simulink model "Scenario_PlusJunction_TrafficLights"  (R2021a)
settings: Solver=VariableStepAuto  StartTime=0.0  StopTime=10.0  RelTol=1e-3
model workspace (MAT data in the model file):
  Kz_dif = Simulink.Parameter
  Kz_dif.Value = Simulink.data.Expression
  Kz_dif.Value.ExpressionString = " L_dif / (Lc + ds)"
  Kz_dif.DataType = 'auto'
  Kz_dif.Dimensions = -1
  Kz_il = Simulink.Parameter
  Kz_il.Value = Simulink.data.Expression
  Kz_il.Value.ExpressionString = " L_il / (Lc + ds)"
  Kz_il.DataType = 'auto'
  Kz_il.Dimensions = -1
  Kz_ir = Simulink.Parameter
  Kz_ir.Value = Simulink.data.Expression
  Kz_ir.Value.ExpressionString = " L_ir / (Lc + ds)"
  Kz_ir.DataType = 'auto'
  Kz_ir.Dimensions = -1
  Kz_is = Simulink.Parameter
  Kz_is.Value = Simulink.data.Expression
  Kz_is.Value.ExpressionString = " L_is / (Lc + ds)"
  Kz_is.DataType = 'auto'
  Kz_is.Dimensions = -1
  Kz_long = Simulink.Parameter
  Kz_long.Value = Simulink.data.Expression
  Kz_long.Value.ExpressionString = " L_long / (Lc + ds)"
  Kz_long.Description = 'Segmentkapazität (wie viele autos passen hinein)'
  Kz_long.DataType = 'auto'
  Kz_long.Dimensions = -1
  Kz_pre = Simulink.Parameter
  Kz_pre.Value = Simulink.data.Expression
  Kz_pre.Value.ExpressionString = " L_pre / (Lc + ds)"
  Kz_pre.DataType = 'auto'
  Kz_pre.Dimensions = -1
  L_dif = Simulink.Parameter
  L_dif.Value = Simulink.data.Expression
  L_dif.Value.ExpressionString = "L_long-L_pre"
  L_dif.Description = 'Differenz zwischen Abbiegerspurlänge und normaler straßenlänge'
  L_dif.DataType = 'auto'
  L_dif.Dimensions = -1
  L_il = Simulink.Parameter
  L_il.Value = 30
  L_il.Description = 'Länge der innenkreuzungssegments, das linksabbieger durchqueren'
  L_il.DataType = 'auto'
  L_il.Dimensions = [1 1]
  L_ir = Simulink.Parameter
  L_ir.Value = 23
  L_ir.Description = 'Länge der innenkreuzungssegments, das rechtsabbieger durchqueren'
  L_ir.DataType = 'auto'
  L_ir.Dimensions = [1 1]
  L_is = Simulink.Parameter
  L_is.Value = 35
  L_is.Description = 'Länge der innenkreuzungssegments, das geradeausfahrer durchqueren'
  L_is.DataType = 'auto'
  L_is.Dimensions = [1 1]
  L_long = Simulink.Parameter
  L_long.Value = 52.8
  L_long.Description = 'Langes straßensegment  (52.8 meter)'
  L_long.DataType = 'auto'
  L_long.Dimensions = [1 1]
  L_pre = Simulink.Parameter
  L_pre.Value = 20
  L_pre.Description = 'Länge der Abbiegespuren'
  L_pre.DataType = 'auto'
  L_pre.Dimensions = [1 1]
  Lc = Simulink.Parameter
  Lc.Value = 4.4
  Lc.Description = 'Länge eines autos'
  Lc.DataType = 'auto'
  Lc.Dimensions = [1 1]
  Rk = Simulink.Parameter
  Rk.Value = Simulink.data.Expression
  Rk.Value.ExpressionString = " 1 / (Lc / v)"
  Rk.Description = 'Flussrate zwischen den Kanten (bei speed v)'
  Rk.DataType = 'auto'
  Rk.Dimensions = -1
  Tz_dif = Simulink.Parameter
  Tz_dif.Value = Simulink.data.Expression
  Tz_dif.Value.ExpressionString = " L_dif / v"
  Tz_dif.DataType = 'auto'
  Tz_dif.Dimensions = -1
  Tz_il = Simulink.Parameter
  Tz_il.Value = Simulink.data.Expression
  Tz_il.Value.ExpressionString = " L_il / v"
  Tz_il.DataType = 'auto'
  Tz_il.Dimensions = -1
  Tz_ir = Simulink.Parameter
  Tz_ir.Value = Simulink.data.Expression
  Tz_ir.Value.ExpressionString = " L_ir / v"
  Tz_ir.DataType = 'auto'
  Tz_ir.Dimensions = -1
  Tz_is = Simulink.Parameter
  Tz_is.Value = Simulink.data.Expression
  Tz_is.Value.ExpressionString = " L_is / v"
  Tz_is.DataType = 'auto'
  Tz_is.Dimensions = -1
  Tz_long = Simulink.Parameter
  Tz_long.Value = Simulink.data.Expression
  Tz_long.Value.ExpressionString = " L_long / v"
  Tz_long.Description = 'Segment durchfahrtzeit: wie lange würde ein auto brauchen,um
    | ungehindert durch das segment zu fahren.'
  Tz_long.DataType = 'auto'
  Tz_long.Dimensions = -1
  Tz_pre = Simulink.Parameter
  Tz_pre.Value = Simulink.data.Expression
  Tz_pre.Value.ExpressionString = " L_pre / v"
  Tz_pre.DataType = 'auto'
  Tz_pre.Dimensions = -1
  ds = Simulink.Parameter
  ds.Value = Simulink.data.Expression
  ds.Value.ExpressionString = "v*dt"
  ds.DataType = 'auto'
  ds.Dimensions = -1
  dt = Simulink.Parameter
  dt.Value = 1
  dt.Description = 'temporaler sicherheitsabstand'
  dt.DataType = 'auto'
  dt.Dimensions = [1 1]
  v = Simulink.Parameter
  v.Value = 13.89
  v.Description = 'geschwindigkeit eines autos
    | (km/h : 3.75 = m/s)
    | 	30km/h = 8,34m/s
    | 	20km/h = 5.56m/s
    | 	50km/h = 13.89m/s
    | '
  v.DataType = 'auto'
  v.Dimensions = [1 1]
libraries: StreetLanesLibrary x32, EdgesLibrary x28, SourcesAndSinksLibrary x8
settings Model: Creator=phill  LastModifiedBy=phill
settings SolverCC: ZeroCrossAlgorithm=Adaptive

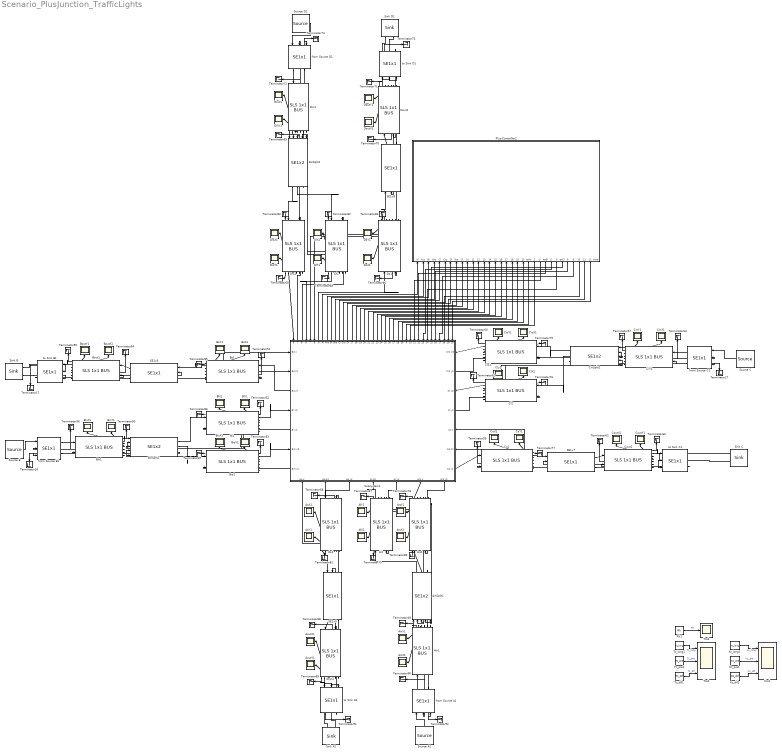
== system Scenario_PlusJunction_TrafficLights ==
  Ain1 : StreetLanesLibrary/SLS 1x1 BUS  Kz=Kz_dif  Tz=Tz_dif
  AinSplit1 : EdgesLibrary/SE1x2  Rk1=0.5*Rk  Rk2=0.5*Rk
  AinX1 : Scope
  AinY1 : Scope
  Al1 : StreetLanesLibrary/SLS 1x1 BUS  Kz=Kz_pre  Tz=Tz_pre
  AlX1 : Scope
  AlY1 : Scope
  Ao1 : StreetLanesLibrary/SLS 1x1 BUS  Kz=Kz_pre  Tz=Tz_pre
  AoX1 : Scope
  AoY1 : Scope
  Aout1 : StreetLanesLibrary/SLS 1x1 BUS  Kz=Kz_dif  Tz=Tz_dif
  AoutX1 : Scope
  AoutY1 : Scope
  Ars1 : StreetLanesLibrary/SLS 1x1 BUS  Kz=Kz_pre  Tz=Tz_pre
  ArsX1 : Scope
  ArsY1 : Scope
  Bin1 : StreetLanesLibrary/SLS 1x1 BUS  Kz=Kz_dif  Tz=Tz_dif
  BinSplit2 : EdgesLibrary/SE1x2  Rk1=0.5*Rk  Rk2=0.5*Rk
  BinX1 : Scope
  BinY1 : Scope
  Bl1 : StreetLanesLibrary/SLS 1x1 BUS  Kz=Kz_pre  Tz=Tz_pre
  BlX1 : Scope
  BlY1 : Scope
  Bo1 : StreetLanesLibrary/SLS 1x1 BUS  Kz=Kz_pre  Tz=Tz_pre
  BoX1 : Scope
  BoY1 : Scope
  Bout1 : StreetLanesLibrary/SLS 1x1 BUS  Kz=Kz_dif  Tz=Tz_dif
  BoutX1 : Scope
  BoutY1 : Scope
  Brs1 : StreetLanesLibrary/SLS 1x1 BUS  Kz=Kz_pre  Tz=Tz_pre
  BrsX1 : Scope
  BrsY1 : Scope
  Cin1 : StreetLanesLibrary/SLS 1x1 BUS  Kz=Kz_dif  Tz=Tz_dif
  CinSplit1 : EdgesLibrary/SE1x2  Rk1=0.5*Rk  Rk2=0.5*Rk
  CinX1 : Scope
  CinY1 : Scope
  Cl1 : StreetLanesLibrary/SLS 1x1 BUS  Kz=Kz_pre  Tz=Tz_pre
  ClX1 : Scope
  Cly1 : Scope
  Co1 : StreetLanesLibrary/SLS 1x1 BUS  Kz=Kz_pre  Tz=Tz_pre
  CoX1 : Scope
  CoY1 : Scope
  Cout1 : StreetLanesLibrary/SLS 1x1 BUS  Kz=Kz_dif  Tz=Tz_dif
  CoutX1 : Scope
  CoutY1 : Scope
  Crs1 : StreetLanesLibrary/SLS 1x1 BUS  Kz=Kz_pre  Tz=Tz_pre
  CrsX1 : Scope
  CrsY1 : Scope
  Din1 : StreetLanesLibrary/SLS 1x1 BUS  Kz=Kz_dif  Tz=Tz_dif
  DinSplit1 : EdgesLibrary/SE1x2  Rk1=0.5*Rk  Rk2=0.5*Rk
  DinX1 : Scope
  DinY1 : Scope
  Dl1 : StreetLanesLibrary/SLS 1x1 BUS  Kz=Kz_pre  Tz=Tz_pre
  DlX1 : Scope
  DlY1 : Scope
  Do1 : StreetLanesLibrary/SLS 1x1 BUS  Kz=Kz_pre  Tz=Tz_pre
  DoX1 : Scope
  DoY1 : Scope
  Dout1 : StreetLanesLibrary/SLS 1x1 BUS  Kz=Kz_dif  Tz=Tz_dif
  DoutX1 : Scope
  DoutY1 : Scope
  Drs1 : StreetLanesLibrary/SLS 1x1 BUS  Kz=Kz_pre  Tz=Tz_pre
  DrsX1 : Scope
  DrsY1 : Scope
  Kz_dif1 : Constant  Value=Kz_dif
  Kz_long1 : Constant  Value=Kz_long
  Kz_pre1 : Constant  Value=Kz_pre
  Kzs1 : Scope  NumInputPorts=3
  Plus-Controller2 : Stateflow chart  TreatAsAtomicUnit=on  mask{green_duration_sr=6, green_duration_l=6, tol=0}
      mask prompts: green_duration_sr "Green Duration for straight/right traffic"; green_duration_l "Green Duration for left traffic"; tol "tolerance"
      settings: PortSchema="{\"entries\":[{\"content\":{\"sides\":[{\"content\":{\"connectorIds\":[]},\"type\":\"ConnectorPlacement.EquallySpacedRectSide\",\"uuid\":\"2590cc03-86a2-4387-8b1b-fdf4c8b68aa6\"},{\"content\":{\"connectorIds\":[],\"side\":\"RIGHT\"},\"type\":\"ConnectorPlacement.EquallySpacedRectSide\",\"uuid\":\"b97063cd-dd31-425f-b4aa-3aaa013ac411\"},{\"content\":{\"connectorIds\":[],\"side\":\"TOP\"},\"type\":\"ConnectorPlacement.EquallySpacedRectSide\",\"uuid\":\"ef5846b9-436e-4b10-a854-1305521b6a0d\"},{\"content\":{\"connectorIds\":[\"In3\",\"In4\",\"In1\",\"In2\",\"In5\",\"In6\",\"In7\",\"In8\",\"In9\",\"In10\",\"In11\",\"In12\",\"In13\",\"In14\",\"In15\",\"In16\",\"In17\",\"In18\",\"In19\",\"In20\",\"Out1\",\"Out2\",\"Out3\",\"Out4\",\"Out5\",\"Out6\",\"Out7\",\"Out8\",\"Out9\",\"Out10\",\"Out11\",\"Out12\",\"Out13\"],\"side\":\"BOTTOM\"},\"type\":\"ConnectorPlacement.EquallySpacedRectSide\",\"uuid\":\"44b73820-3b7c-4ee5-b5da-9465e85a924e\"}]},\"type\":\"ConnectorPlacement.EquallySpacedConnector\",\"uuid\":\"3342797d-7762-4a2a-891a-654024402a66\"}],\"packageUris\":[\"http://schema.mathworks.com/mf0/Connector/R2020b\"],\"version\":\"1.0\"}"
  Rk1 : Constant  Value=Rk
  SE1x{5..8} (4 alike) : EdgesLibrary/SE1x1  Rk=Rk  slope=2000
  Sink A1 : SourcesAndSinksLibrary/Sink  SystemSampleTime=-1  VariantActivationTime=update diagram  Latency=0  AutoFrameSizeCalculation=off
      settings: PortSchema="{\"entries\":[{\"content\":{\"sides\":[{\"content\":{\"connectorIds\":[\"Out1\",\"Out2\"]},\"type\":\"ConnectorPlacement.EquallySpacedRectSide\",\"uuid\":\"9fd2383e-3590-4f0f-bafc-5a4adfbb32b4\"},{\"content\":{\"connectorIds\":[],\"side\":\"RIGHT\"},\"type\":\"ConnectorPlacement.EquallySpacedRectSide\",\"uuid\":\"1e687aa9-1098-45bd-a1f6-ea403f3f2897\"},{\"content\":{\"connectorIds\":[],\"side\":\"TOP\"},\"type\":\"ConnectorPlacement.EquallySpacedRectSide\",\"uuid\":\"fe6eaa71-085c-414b-983a-a0e72e52a49c\"}]},\"type\":\"ConnectorPlacement.EquallySpacedConnector\",\"uuid\":\"370c1712-4373-4726-99c2-6cb04807ece1\"}],\"packageUris\":[\"http://schema.mathworks.com/mf0/Connector/R2020b\"],\"version\":\"1.0\"}"
  Sink B : SourcesAndSinksLibrary/Sink  SystemSampleTime=-1  VariantActivationTime=update diagram  Latency=0  AutoFrameSizeCalculation=off
      settings: PortSchema="{\"entries\":[{\"content\":{\"sides\":[{\"content\":{\"connectorIds\":[\"Out1\",\"Out2\"]},\"type\":\"ConnectorPlacement.EquallySpacedRectSide\",\"uuid\":\"9fd2383e-3590-4f0f-bafc-5a4adfbb32b4\"},{\"content\":{\"connectorIds\":[],\"side\":\"RIGHT\"},\"type\":\"ConnectorPlacement.EquallySpacedRectSide\",\"uuid\":\"1e687aa9-1098-45bd-a1f6-ea403f3f2897\"},{\"content\":{\"connectorIds\":[],\"side\":\"TOP\"},\"type\":\"ConnectorPlacement.EquallySpacedRectSide\",\"uuid\":\"fe6eaa71-085c-414b-983a-a0e72e52a49c\"}]},\"type\":\"ConnectorPlacement.EquallySpacedConnector\",\"uuid\":\"370c1712-4373-4726-99c2-6cb04807ece1\"}],\"packageUris\":[\"http://schema.mathworks.com/mf0/Connector/R2020b\"],\"version\":\"1.0\"}"
  Sink C : SourcesAndSinksLibrary/Sink  SystemSampleTime=-1  VariantActivationTime=update diagram  Latency=0  AutoFrameSizeCalculation=off
      settings: PortSchema="{\"entries\":[{\"content\":{\"sides\":[{\"content\":{\"connectorIds\":[\"Out1\",\"Out2\"]},\"type\":\"ConnectorPlacement.EquallySpacedRectSide\",\"uuid\":\"9fd2383e-3590-4f0f-bafc-5a4adfbb32b4\"},{\"content\":{\"connectorIds\":[],\"side\":\"RIGHT\"},\"type\":\"ConnectorPlacement.EquallySpacedRectSide\",\"uuid\":\"1e687aa9-1098-45bd-a1f6-ea403f3f2897\"},{\"content\":{\"connectorIds\":[],\"side\":\"TOP\"},\"type\":\"ConnectorPlacement.EquallySpacedRectSide\",\"uuid\":\"fe6eaa71-085c-414b-983a-a0e72e52a49c\"}]},\"type\":\"ConnectorPlacement.EquallySpacedConnector\",\"uuid\":\"370c1712-4373-4726-99c2-6cb04807ece1\"}],\"packageUris\":[\"http://schema.mathworks.com/mf0/Connector/R2020b\"],\"version\":\"1.0\"}"
  Sink D1 : SourcesAndSinksLibrary/Sink  SystemSampleTime=-1  VariantActivationTime=update diagram  Latency=0  AutoFrameSizeCalculation=off
      settings: PortSchema="{\"entries\":[{\"content\":{\"sides\":[{\"content\":{\"connectorIds\":[\"Out1\",\"Out2\"]},\"type\":\"ConnectorPlacement.EquallySpacedRectSide\",\"uuid\":\"9fd2383e-3590-4f0f-bafc-5a4adfbb32b4\"},{\"content\":{\"connectorIds\":[],\"side\":\"RIGHT\"},\"type\":\"ConnectorPlacement.EquallySpacedRectSide\",\"uuid\":\"1e687aa9-1098-45bd-a1f6-ea403f3f2897\"},{\"content\":{\"connectorIds\":[],\"side\":\"TOP\"},\"type\":\"ConnectorPlacement.EquallySpacedRectSide\",\"uuid\":\"fe6eaa71-085c-414b-983a-a0e72e52a49c\"}]},\"type\":\"ConnectorPlacement.EquallySpacedConnector\",\"uuid\":\"370c1712-4373-4726-99c2-6cb04807ece1\"}],\"packageUris\":[\"http://schema.mathworks.com/mf0/Connector/R2020b\"],\"version\":\"1.0\"}"
  Source A1 : SourcesAndSinksLibrary/Source  SystemSampleTime=-1  VariantActivationTime=update diagram  Latency=0  AutoFrameSizeCalculation=off
  Source B : SourcesAndSinksLibrary/Source  SystemSampleTime=-1  VariantActivationTime=update diagram  Latency=0  AutoFrameSizeCalculation=off
  Source C : SourcesAndSinksLibrary/Source  SystemSampleTime=-1  VariantActivationTime=update diagram  Latency=0  AutoFrameSizeCalculation=off
  Source D1 : SourcesAndSinksLibrary/Source  SystemSampleTime=-1  VariantActivationTime=update diagram  Latency=0  AutoFrameSizeCalculation=off
  Subsystem1 : Subsystem  mask{Kz_left=Kz_il, Tz_left=Tz_il, Kz_straight=Kz_is, Tz_straight=Tz_is, Kz_right=Kz_ir, Tz_right=Tz_ir, Rk=Rk}
      settings: PortSchema="{\"entries\":[{\"content\":{\"sides\":[{\"content\":{\"connectorIds\":[\"In1\",\"In2\",\"Out30\",\"In3\",\"Out31\",\"In4\",\"Out32\"]},\"type\":\"ConnectorPlacement.EquallySpacedRectSide\",\"uuid\":\"223afcc5-5490-41e2-b2c1-0ac31bdd31f0\"},{\"content\":{\"connectorIds\":[\"In25\",\"Out1\",\"In26\",\"Out2\",\"In27\",\"In28\",\"Out3\"],\"side\":\"RIGHT\"},\"type\":\"ConnectorPlacement.EquallySpacedRectSide\",\"uuid\":\"e803e5ea-345a-49fc-8782-ffb100729ba0\"},{\"content\":{\"connectorIds\":[\"In5\",\"Out7\",\"Out8\",\"In6\",\"In7\",\"In8\",\"Out9\",\"Out10\",\"Out11\",\"Out12\",\"Out13\",\"Out14\",\"Out15\",\"Out16\",\"Out17\",\"Out18\",\"Out19\",\"Out20\",\"Out21\",\"Out22\",\"Out23\",\"Out24\",\"Out25\",\"Out26\",\"Out27\",\"Out28\",\"Out29\",\"In9\",\"In10\",\"In11\",\"In12\",\"In13\",\"In14\",\"In15\",\"In16\",\"In17\",\"In18\",\"In19\",\"In20\"],\"side\":\"TOP\"},\"type\":\"ConnectorPlacement.EquallySpacedRectSide\",\"uuid\":\"8581fbf9-6742-4a7a-9e93-ed29b1a56c31\"},{\"content\":{\"connectorIds\":[\"In21\",\"In22\",\"Out4\",\"In23\",\"Out5\",\"In24\",\"Out6\"],\"side\":\"BOTTOM\"},\"type\":\"ConnectorPlacement.EquallySpacedRectSide\",\"uuid\":\"cc67de78-9dd9-463d-9445-caa2eb7c099b\"}]},\"type\":\"ConnectorPlacement.EquallySpacedConnector\",\"uuid\":\"ac6fc4cc-2326-4bcf-896c-a5d089a8f47a\"}],\"packageUris\":[\"http://schema.mathworks.com/mf0/Connector/R2020b\"],\"version\":\"1.0\"}"
      mask Display:
      | %image('$imagefile'); % Use "Edit Image" on toolstrip to change.
      | disp('+ \n\n');
      | KzS = get_param(gcb,'Kz_straight');
      | TzS = get_param(gcb,'Tz_straight');
      | KzR = get_param(gcb,'Kz_right');
      | TzR = get_param(gcb,'Tz_right');
      | KzL = get_param(gcb,'Kz_left');
      | TzL = get_param(gcb,'Tz_left');
      | Rk = get_param(gcb,'Rk');
      | disp(['Rk = ', Rk, ' | Kz/Tz L = ', KzL, ' ', TzL, ' | Kz/Tz S = ', KzS, ' ', TzS, ' | Kz/Tz R = ', KzR, ' ', TzR]);
  Terminator{17..18,27,49..92} (47 alike) : Terminator
  Tz_dif1 : Constant  Value=Tz_dif
  Tz_long1 : Constant  Value=Tz_long
  Tz_pre1 : Constant  Value=Tz_pre
  Tzs2 : Scope  NumInputPorts=3
  Tzs3 : Scope
  from Source A1 : EdgesLibrary/SE1x1  Rk=Rk  slope=2000
  from Source B1 : EdgesLibrary/SE1x1  Rk=Rk  slope=2000
  from Source C1 : EdgesLibrary/SE1x1  Rk=Rk  slope=2000
  from Source D1 : EdgesLibrary/SE1x1  Rk=Rk  slope=2000
  to Sink A1 : EdgesLibrary/SE1x1  Rk=Rk  slope=2000
  to Sink B1 : EdgesLibrary/SE1x1  Rk=Rk  slope=2000
  to Sink C1 : EdgesLibrary/SE1x1  Rk=Rk  slope=2000
  to Sink D1 : EdgesLibrary/SE1x1  Rk=Rk  slope=2000
  wires:
  Source B/1 -> from Source B1/1
  to Sink B1/1 -> Terminator17/1
  from Source B1/2 -> Terminator18/1
  Sink B/1 -> to Sink B1/2
  Sink B/2 -> to Sink B1/3
  Source C/1 -> from Source C1/1
  Cout1/1 -> Terminator63/1
  Crs1/6 -> CinSplit1/2
  SE1x5/2 -> Ao1/2
  Bl1/1 -> Terminator52/1
  SE1x8/1 -> Dout1/1
  to Sink D1/2 -> Dout1/2
  from Source C1/1 -> Cin1/1
  Tz_dif1/1 -> Tzs2/3  "Tz_dif"
  Dl1/1 -> Terminator68/1
  Subsystem1/30(Bo yk) -> Bo1/1
  from Source C1/2 -> Terminator27/1
  Crs1/3 -> CrsX1/1
  to Sink A1/1 -> Terminator91/1
  Din1/6 -> from Source D1/2
  Sink C/1 -> to Sink C1/2
  Drs1/5 -> Terminator83/1
  Ao1/6 -> Subsystem1/21(Ao x)
  Aout1/2 -> to Sink A1/1
  Dl1/4 -> DlY1/1
  Co1/1 -> Terminator77/1
  CinSplit1/2 -> Cl1/1
  AinSplit1/2 -> Ars1/1
  Ain1/2 -> AinSplit1/1
  Crs1/7 -> CinSplit1/3
  BinSplit2/2 -> Brs1/1
  Sink D1/1 -> to Sink D1/2
  Al1/5 -> Terminator79/1
  Bo1/1 -> Terminator85/1
  Kz_dif1/1 -> Kzs1/3  "Kz_dif"
  Bin1/5 -> Terminator56/1
  Cout1/2 -> to Sink C1/1
  Subsystem1/6(Ars yk) -> Ars1/2
  Cout1/4 -> CoutY1/1
  Drs1/1 -> Terminator69/1
  Brs1/4 -> BrsY1/1
  CinSplit1/1 -> Crs1/1
  Subsystem1/4(Ao yk) -> Ao1/1
  Drs1/7 -> DinSplit1/3
  Din1/7 -> from Source D1/3
  Dout1/7 -> SE1x8/3
  Drs1/2 -> Subsystem1/5(Drs x0)
  Cl1/5 -> Terminator76/1
  Dout1/3 -> DoutX1/1
  Drs1/6 -> DinSplit1/2
  CinSplit1/3 -> Cin1/2
  Ao1/2 -> SE1x5/1
  Bout1/3 -> BoutX1/1
  Subsystem1/32(Brs yk) -> Brs1/2
  Brs1/1 -> Terminator53/1
  Cl1/4 -> Cly1/1
  Do1/7 -> Subsystem1/8(Do Kz)
  Cl1/3 -> ClX1/1
  Bl1/5 -> Terminator86/1
  Subsystem1/3(Co yk) -> Co1/1
  Sink A1/2 -> to Sink A1/3
  Ars1/5 -> Terminator80/1
  DinSplit1/3 -> Din1/2
  Dout1/6 -> SE1x8/2
  Bout1/5 -> Terminator54/1
  Bout1/2 -> to Sink B1/1
  Ars1/2 -> Subsystem1/24(Ars x)
  Cout1/3 -> CoutX1/1
  Dl1/3 -> DlX1/1
  from Source D1/1 -> Din1/1
  Sink A1/1 -> to Sink A1/2
  Co1/7 -> Subsystem1/28(Co Kz)
  Dl1/7 -> DinSplit1/5
  Subsystem1/2(Cl yk) -> Cl1/2
  Co1/3 -> CoX1/1
  Bout1/1 -> Terminator55/1
  Do1/5 -> Terminator66/1
  Al1/2 -> Subsystem1/23(Al x0)
  Bout1/4 -> BoutY1/1
  BinSplit2/1 -> Bl1/1
  Brs1/2 -> Subsystem1/4(Brs x0)
  Bin1/4 -> BinY1/1
  SE1x6/2 -> Bo1/2
  SE1x5/1 -> Aout1/1
  Crs1/1 -> Terminator60/1
  Subsystem1/31(Bl yk) -> Bl1/2
  Brs1/7 -> BinSplit2/5
  Dl1/6 -> DinSplit1/4
  Do1/2 -> SE1x8/1
  Dout1/4 -> DoutY1/1
  Al1/7 -> AinSplit1/3
  Bin1/7 -> from Source B1/3
  Din1/1 -> Terminator65/1
  Cl1/7 -> CinSplit1/5
  Bin1/3 -> BinX1/1
  Dl1/5 -> Terminator82/1
  from Source D1/2 -> Terminator74/1
  DinSplit1/1 -> Drs1/1
  SE1x6/1 -> Bout1/1
  to Sink C1/2 -> Cout1/2
  Tz_pre1/1 -> Tzs2/2  "Tz_pre"
  Do1/4 -> DoY1/1
  Cin1/5 -> Terminator64/1
  Cin1/6 -> from Source C1/2
  Bout1/6 -> SE1x6/2
  Subsystem1/1(Crs yk) -> Crs1/2
  Ars1/4 -> ArsY1/1
  Al1/3 -> AlX1/1
  Al1/4 -> AlY1/1
  Ain1/7 -> from Source A1/3
  Kz_long1/1 -> Kzs1/1  "Kz_long"
  Ao1/1 -> Terminator81/1
  Bout1/7 -> SE1x6/3
  Tz_long1/1 -> Tzs2/1  "Tz_long"
  Cout1/5 -> Terminator62/1
  Brs1/5 -> Terminator87/1
  AinSplit1/3 -> Ain1/2
  Cl1/6 -> CinSplit1/4
  SE1x7/1 -> Cout1/1
  Cout1/7 -> SE1x7/3
  Bo1/4 -> BoY1/1
  Cin1/7 -> from Source C1/3
  Aout1/3 -> AoutX1/1
  Ain1/5 -> Terminator90/1
  Al1/6 -> AinSplit1/2
  Subsystem1/9(Do yk) -> Do1/1
  Ars1/6 -> AinSplit1/4
  Din1/5 -> Terminator72/1
  Bin1/6 -> from Source B1/2
  Cin1/3 -> CinX1/1
  Source A1/1 -> from Source A1/1
  Cin1/2 -> CinSplit1/1
  from Source A1/1 -> Ain1/1
  Ain1/4 -> AinY1/1
  Ao1/3 -> AoX1/1
  Bl1/3 -> BlX1/1
  Dout1/1 -> Terminator71/1
  Bo1/2 -> SE1x6/1
  Aout1/6 -> SE1x5/2
  Ain1/6 -> from Source A1/2
  Crs1/2 -> Subsystem1/25(Crs x0)
  Brs1/3 -> BrsX1/1
  DinSplit1/2 -> Dl1/1
  SE1x7/2 -> Co1/2
  Plus-Controller2/10(enDl) -> Subsystem1/18(enDl)
  Cl1/2 -> Subsystem1/26(Cl x0)
  Drs1/4 -> DrsY1/1
  Plus-Controller2/11(enDs) -> Subsystem1/19(enDs)
  Ars1/7 -> AinSplit1/5
  Subsystem1/11(Ars) -> Plus-Controller2/4(Ars)
  Subsystem1/22(Brs_Co) -> Plus-Controller2/13(Brs_Co)
  Ao1/7 -> Subsystem1/22(Ao Kz)
  Subsystem1/20(Ars_Co) -> Plus-Controller2/11(Ars_Co)
  Subsystem1/24(Cl_Ao) -> Plus-Controller2/15(Cl_Ao)
  Bo1/5 -> Terminator51/1
  Brs1/6 -> BinSplit2/4
  Co1/2 -> SE1x7/1
  Plus-Controller2/3(enAr) -> Subsystem1/11(enAr)
  Al1/1 -> Terminator67/1
  Bl1/4 -> BlY1/1
  Bo1/3 -> BoX1/1
  Plus-Controller2/12(enDr) -> Subsystem1/20(enDr)
  Co1/5 -> Terminator59/1
  Cin1/4 -> CinY1/1
  BinSplit2/3 -> Bin1/2
  Plus-Controller2/9(enCr) -> Subsystem1/17(enCr)
  Subsystem1/7(Drs yk) -> Drs1/2
  Drs1/3 -> DrsX1/1
  SE1x8/2 -> Do1/2
  Plus-Controller2/8(enCs) -> Subsystem1/16(enCs)
  Subsystem1/28(Drs_Ao) -> Plus-Controller2/19(Drs_Ao)
  Plus-Controller2/4(enBl) -> Subsystem1/12(enBl)
  Bl1/2 -> Subsystem1/3(Bl x0)
  from Source A1/2 -> Terminator92/1
  Subsystem1/19(Ars_Do) -> Plus-Controller2/10(Ars_Do)
  Kz_pre1/1 -> Kzs1/2  "Kz_pre"
  Plus-Controller2/2(enAs) -> Subsystem1/10(enAs)
  Do1/6 -> Subsystem1/7(Do x)
  Din1/4 -> DinY1/1
  Plus-Controller2/5(enBs) -> Subsystem1/13(enBs)
  Plus-Controller2/6(enBr) -> Subsystem1/14(enBr)
  Subsystem1/27(Dl_Co) -> Plus-Controller2/18(Dl_Co)
  Subsystem1/25(Crs_Bo) -> Plus-Controller2/16(Crs_Bo)
  Subsystem1/23(Brs_Ao) -> Plus-Controller2/14(Brs_Ao)
  Subsystem1/5(Al yk) -> Al1/2
  Aout1/5 -> Terminator88/1
  Plus-Controller2/7(enCl) -> Subsystem1/15(enCl)
  Subsystem1/26(Crs_Do) -> Plus-Controller2/17(Crs_Do)
  Subsystem1/12(Bl) -> Plus-Controller2/1(Bl)
  Crs1/5 -> Terminator75/1
  Subsystem1/17(Drs) -> Plus-Controller2/8(Drs)
  Dl1/2 -> Subsystem1/6(Dl x0)
  to Sink A1/2 -> Aout1/2
  Subsystem1/18(Al_Bo) -> Plus-Controller2/9(Al_Bo)
  Cout1/6 -> SE1x7/2
  Do1/3 -> DoX1/1
  Co1/6 -> Subsystem1/27(Co x)
  Subsystem1/15(Crs) -> Plus-Controller2/6(Crs)
  Ao1/4 -> AoY1/1
  from Source B1/1 -> Bin1/1
  Aout1/7 -> SE1x5/3
  Cin1/1 -> Terminator57/1
  Bo1/7 -> Subsystem1/2(Bo Kz)
  Din1/3 -> DinX1/1
  Ao1/5 -> Terminator58/1
  Subsystem1/14(Cl) -> Plus-Controller2/5(Cl)
  Bo1/6 -> Subsystem1/1(Bo x)
  Subsystem1/13(Brs) -> Plus-Controller2/2(Brs)
  Subsystem1/10(Al) -> Plus-Controller2/3(Al)
  Sink C/2 -> to Sink C1/3
  Ars1/3 -> ArsX1/1
  to Sink B1/2 -> Bout1/2
  Subsystem1/29(Drs_Bo) -> Plus-Controller2/20(Drs_Bo)
  Cl1/1 -> Terminator61/1
  AinSplit1/1 -> Al1/1
  Co1/4 -> CoY1/1
  Dout1/2 -> to Sink D1/1
  Aout1/4 -> AoutY1/1
  Sink D1/2 -> to Sink D1/3
  Subsystem1/8(Dl yk) -> Dl1/2
  Bin1/1 -> Terminator50/1
  Din1/2 -> DinSplit1/1
  to Sink D1/1 -> Terminator73/1
  Subsystem1/21(Bl_Do) -> Plus-Controller2/12(Bl_Do)
  Ain1/1 -> Terminator49/1
  Aout1/1 -> Terminator89/1
  Crs1/4 -> CrsY1/1
  Rk1/1 -> Tzs3/1  "Rk"
  Bl1/6 -> BinSplit2/2
  Bin1/2 -> BinSplit2/1
  Bl1/7 -> BinSplit2/3
  Do1/1 -> Terminator84/1
  Source D1/1 -> from Source D1/1
  Ain1/3 -> AinX1/1
  Dout1/5 -> Terminator70/1
  Plus-Controller2/1(enAl) -> Subsystem1/9(enAl)
  Ars1/1 -> Terminator78/1
  Subsystem1/16(Dl) -> Plus-Controller2/7(Dl)

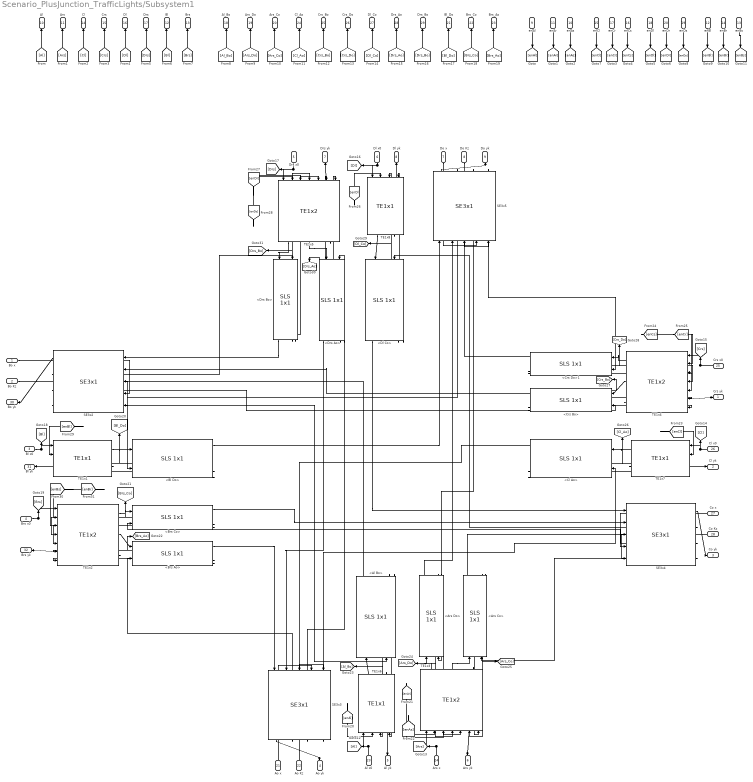
== system Scenario_PlusJunction_TrafficLights/Subsystem1 ==
  Bo x : Inport
  Bo Kz : Inport  Port=2
  Bl x0 : Inport  Port=3
  Brs x0 : Inport  Port=4
  Drs x0 : Inport  Port=5
  Dl x0 : Inport  Port=6
  Do x : Inport  Port=7
  Do Kz : Inport  Port=8
  enAl : Inport  Port=9
  enAs : Inport  Port=10
  enAr : Inport  Port=11
  enBl : Inport  Port=12
  enBs : Inport  Port=13
  enBr : Inport  Port=14
  enCl : Inport  Port=15
  enCs : Inport  Port=16
  enCr : Inport  Port=17
  enDl : Inport  Port=18
  enDs : Inport  Port=19
  enDr : Inport  Port=20
  Ao x : Inport  Port=21
  Ao Kz : Inport  Port=22
  Al x0 : Inport  Port=23
  Ars x : Inport  Port=24
  Crs x0 : Inport  Port=25
  Cl x0 : Inport  Port=26
  Co x : Inport  Port=27
  Co Kz : Inport  Port=28
  <Al Bo> : StreetLanesLibrary/SLS 1x1  Kz=Kz_left  Tz=Tz_left
  <Ars Co> : StreetLanesLibrary/SLS 1x1  Kz=Kz_right  Tz=Tz_right
  <Ars Do> : StreetLanesLibrary/SLS 1x1  Kz=Kz_straight  Tz=Tz_straight
  <Bl Do> : StreetLanesLibrary/SLS 1x1  Kz=Kz_left  Tz=Tz_left
  <Brs Ao> : StreetLanesLibrary/SLS 1x1  Kz=Kz_right  Tz=Tz_right
  <Brs Co> : StreetLanesLibrary/SLS 1x1  Kz=Kz_straight  Tz=Tz_straight
  <Cl Ao> : StreetLanesLibrary/SLS 1x1  Kz=Kz_left  Tz=Tz_left
  <Crs Bo> : StreetLanesLibrary/SLS 1x1  Kz=Kz_straight  Tz=Tz_straight
  <Crs Do>1 : StreetLanesLibrary/SLS 1x1  Kz=Kz_right  Tz=Tz_right
  <Dl Co> : StreetLanesLibrary/SLS 1x1  Kz=Kz_left  Tz=Tz_left
  <Drs Ao> : StreetLanesLibrary/SLS 1x1  Kz=Kz_straight  Tz=Tz_straight
  <Drs Bo> : StreetLanesLibrary/SLS 1x1  Kz=Kz_right  Tz=Tz_right
  SE3x{2..5} (4 alike) : EdgesLibrary/SE3x1  Rk1=Rk  Rk2=Rk  Rk3=Rk
  TE1x{1,6..8} (4 alike) : EdgesLibrary/TE1x1  Rk=Rk  slope=2000
  TE1x{2..5} (4 alike) : EdgesLibrary/TE1x2  Rk1=0.5*Rk  Rk2=0.5*Rk
  Crs yk : Outport
  Cl yk : Outport  Port=2
  Co yk : Outport  Port=3
  Ao yk : Outport  Port=4
  Al yk : Outport  Port=5
  Ars yk : Outport  Port=6
  Drs yk : Outport  Port=7
  Dl yk : Outport  Port=8
  Do yk : Outport  Port=9
  Al : Outport  Port=10
  Ars : Outport  Port=11
  Bl : Outport  Port=12
  Brs : Outport  Port=13
  Cl : Outport  Port=14
  Crs : Outport  Port=15
  Dl : Outport  Port=16
  Drs : Outport  Port=17
  Al_Bo : Outport  Port=18
  Ars_Do : Outport  Port=19
  Ars_Co : Outport  Port=20
  Bl_Do : Outport  Port=21
  Brs_Co : Outport  Port=22
  Brs_Ao : Outport  Port=23
  Cl_Ao : Outport  Port=24
  Crs_Bo : Outport  Port=25
  Crs_Do : Outport  Port=26
  Dl_Co : Outport  Port=27
  Drs_Ao : Outport  Port=28
  Drs_Bo : Outport  Port=29
  Bo yk : Outport  Port=30
  Bl yk : Outport  Port=31
  Brs yk : Outport  Port=32
  wires:
  SE3x2/1 -> Bo yk/1
  Bo Kz/1 -> SE3x2/5
  Bo x/1 -> SE3x2/4
  Bl x0/1 -> [Bl], TE1x1/1
  TE1x1/2 -> Bl yk/1
  Brs x0/1 -> [Brs], TE1x2/1
  TE1x2/3 -> Brs yk/1
  Ao x/1 -> SE3x3/4
  Ao Kz/1 -> SE3x3/5
  SE3x3/1 -> Ao yk/1
  Ars x/1 -> [Ars], TE1x3/1
  TE1x3/3 -> Ars yk/1
  Co Kz/1 -> SE3x4/5
  Co x/1 -> SE3x4/4
  SE3x4/1 -> Co yk/1
  TE1x4/3 -> Crs yk/1
  Crs x0/1 -> [Crs], TE1x4/1
  Do x/1 -> SE3x5/4
  Do Kz/1 -> SE3x5/5
  SE3x5/1 -> Do yk/1
  TE1x5/3 -> Drs yk/1
  Drs x0/1 -> [Drs], TE1x5/1
  TE1x4/2 -> <Crs Bo>/1
  <Crs Bo>/8 -> TE1x4/7
  <Crs Bo>/7 -> [Crs_Bo], TE1x4/6
  TE1x3/1 -> <Ars Do>/1
  <Ars Do>/8 -> TE1x3/5
  <Ars Do>/7 -> [Ars_Do], TE1x3/4
  TE1x2/1 -> <Brs Co>/1
  <Brs Co>/8 -> TE1x2/5
  <Brs Co>/7 -> [Brs_Co], TE1x2/4
  TE1x2/2 -> <Brs Ao>/1
  <Brs Ao>/8 -> TE1x2/7
  <Brs Ao>/7 -> TE1x2/6, [Brs_Ao]
  TE1x4/1 -> <Crs Do>1/1
  <Crs Do>1/8 -> TE1x4/5
  <Crs Do>1/7 -> [Crs_Do], TE1x4/4
  TE1x5/1 -> <Drs Bo>/1
  <Drs Bo>/8 -> TE1x5/5
  TE1x5/2 -> <Drs Ao>/1
  <Drs Ao>/8 -> TE1x5/7
  <Drs Ao>/7 -> [Drs_Ao], TE1x5/6
  TE1x3/2 -> <Ars Co>/1
  <Ars Co>/8 -> TE1x3/7
  TE1x1/1 -> <Bl Do>/1
  <Bl Do>/8 -> TE1x1/4
  <Bl Do>/7 -> [Bl_Do], TE1x1/3
  <Cl Ao>/7 -> TE1x7/3, [Cl_Ao]
  <Cl Ao>/8 -> TE1x7/4
  TE1x7/1 -> <Cl Ao>/1
  TE1x8/1 -> <Dl Co>/1
  <Dl Co>/8 -> TE1x8/4
  <Dl Co>/7 -> [Dl_Co], TE1x8/3
  TE1x6/1 -> <Al Bo>/1
  <Al Bo>/8 -> TE1x6/4
  <Al Bo>/7 -> TE1x6/3, [Al_Bo]
  <Drs Bo>/2 -> SE3x2/1
  SE3x2/2 -> <Drs Bo>/2
  <Crs Bo>/2 -> SE3x2/2
  SE3x2/3 -> <Crs Bo>/2
  <Al Bo>/2 -> SE3x2/3
  SE3x2/4 -> <Al Bo>/2
  <Crs Do>1/2 -> SE3x5/3
  SE3x5/4 -> <Crs Do>1/2
  SE3x5/3 -> <Ars Do>/2
  <Ars Do>/2 -> SE3x5/2
  <Bl Do>/2 -> SE3x5/1
  SE3x5/2 -> <Bl Do>/2
  SE3x4/4 -> <Ars Co>/2
  <Ars Co>/2 -> SE3x4/3
  SE3x4/3 -> <Brs Co>/2
  <Brs Co>/2 -> SE3x4/2
  SE3x4/2 -> <Dl Co>/2
  <Dl Co>/2 -> SE3x4/1
  SE3x3/2 -> <Brs Ao>/2
  <Brs Ao>/2 -> SE3x3/1
  SE3x3/3 -> <Drs Ao>/2
  <Drs Ao>/2 -> SE3x3/2
  SE3x3/4 -> <Cl Ao>/2
  <Cl Ao>/2 -> SE3x3/3
  <Ars Co>/7 -> TE1x3/6, [Ars_Co]
  Al x0/1 -> [Al], TE1x6/1
  TE1x6/2 -> Al yk/1
  Cl x0/1 -> [Cl], TE1x7/1
  TE1x7/2 -> Cl yk/1
  Dl x0/1 -> [Dl], TE1x8/1
  TE1x8/2 -> Dl yk/1
  [enAl] -> TE1x6/2
  [enAr] -> TE1x3/3
  [enAs] -> TE1x3/2
  [enCl] -> TE1x7/2
  [enCs] -> TE1x4/3
  [enCr] -> TE1x4/2
  [enDl] -> TE1x8/2
  [enBl] -> TE1x1/2
  [enBs] -> TE1x2/2
  [enBr] -> TE1x2/3
  [enDr] -> TE1x5/2
  [enDs] -> TE1x5/3
  <Drs Bo>/7 -> TE1x5/4, [Drs_Bo]
  [Al] -> Al/1
  [Ars] -> Ars/1
  [Cl] -> Cl/1
  [Crs] -> Crs/1
  [Dl] -> Dl/1
  [Drs] -> Drs/1
  [Bl] -> Bl/1
  [Brs] -> Brs/1
  [Al_Bo] -> Al_Bo/1
  [Ars_Do] -> Ars_Do/1
  [Ars_Co] -> Ars_Co/1
  [Cl_Ao] -> Cl_Ao/1
  [Crs_Bo] -> Crs_Bo/1
  [Crs_Do] -> Crs_Do/1
  [Dl_Co] -> Dl_Co/1
  [Drs_Ao] -> Drs_Ao/1
  [Drs_Bo] -> Drs_Bo/1
  [Bl_Do] -> Bl_Do/1
  [Brs_Co] -> Brs_Co/1
  [Brs_Ao] -> Brs_Ao/1
  enAl/1 -> [enAl]
  enAr/1 -> [enAr]
  enAs/1 -> [enAs]
  enCl/1 -> [enCl]
  enCr/1 -> [enCr]
  enCs/1 -> [enCs]
  enDl/1 -> [enDl]
  enDr/1 -> [enDr]
  enDs/1 -> [enDs]
  enBl/1 -> [enBl]
  enBr/1 -> [enBr]
  enBs/1 -> [enBs]

== stateflow chart Scenario_PlusJunction_TrafficLights/Plus-Controller2 ==
  state CompleteController
    state timecounter [parallel]
      settings: executionOrder=1
    state actualController [parallel]
      settings: executionOrder=2
      (history)
      note: ?
      state Group__Crs_Brs
      state Group__Cl_Bl
      state Group__Ars_Drs
      state Group__Al_Dl
      note: check
          | Crs straight
          | crossings
      note: check
          | Cl
          | crossings
      note: check
          | Ars straight
          | crossings
      note: check
          | Al
          | crossings
      note: check
          | Crs right
          | crossings
      note: check
          | Bl
          | crossings
      note: check
          | Ars right
          | crossings
      note: check
          | Dl
          | crossings
      note: check
          | Brs straight
          | crossings
      note: check
          | Drs straight
          | crossings
      note: check
          | Brs right
          | crossings
      note: check
          | Drs right
          | crossings
      Group__Al_Dl -> Group__Crs_Brs [order 1] : [time >= green_duration_l]
          | {enAl = 0; enDl = 0; time = 0;}
      Group__Ars_Drs -> Group__Al_Dl [order 1] : [time >=green_duration_sr]
          | {enAs = 0; enAr = 0; enDs = 0; enDr = 0; time = 0;}
      Group__Cl_Bl -> Group__Ars_Drs [order 1] : [time >= green_duration_l]
          | {enCl = 0; enBl = 0; time = 0;}
      Group__Crs_Brs -> Group__Cl_Bl [order 1] : [time >= green_duration_sr]
          | {enCs = 0; enCr = 0; enBs = 0;
          | enBr = 0; time = 0;}
      (default) -> Group__Crs_Brs : {enAl = 0; enAs = 0; enAr = 0;
          | enBl = 0; enBs = 0; enBr = 0;
          | enCl = 0; enCs = 0; enCr = 0;
          | enDl = 0; enDs = 0; enDr = 0;}
      Group__Crs_Brs -> (junction 51) [order 2]
      (junction 109) -> Group__Crs_Brs
      Group__Cl_Bl -> (junction 117) [order 2]
      (junction 126) -> Group__Cl_Bl
      Group__Ars_Drs -> (junction 134) [order 2]
      (junction 131) -> Group__Ars_Drs
      Group__Al_Dl -> (junction 151) [order 2]
      (junction 160) -> Group__Al_Dl
      (junction 117) -> (junction 116) [order 2] : {enCl = 0;}
      (junction 51) -> (junction 59) [order 1] : [(Dl_Co<=tol && Drs_Ao<=tol ...
          | && Drs_Bo<=tol && Bl_Do<=tol ...
          | && Al_Bo<=tol && Ars_Do<=tol)]
          | {enCs = 1;}
      (junction 117) -> (junction 116) [order 1] : [Dl_Co<=tol && Drs_Ao<=tol && ....
          | Brs_Co<=tol && Al_Bo<=tol && ...
          | Ars_Do<=tol && Brs_Ao]{enCl = 1;}
      (junction 51) -> (junction 59) [order 2] : {enCs = 0;}
      (junction 134) -> (junction 133) [order 1] : [Cl_Ao<=tol && Crs_Bo<=tol && ...
          | Crs_Do<=tol && Dl_Co<=tol && ...
          | Bl_Do<=tol && Brs_Co<=tol]
          | {enAs = 1;}
      (junction 151) -> (junction 150) [order 1] : [(Cl_Ao<=tol && Crs_Bo<=tol ...
          | && Drs_Ao<=tol && Bl_Do<=tol ...
          | && Brs_Co<=tol && Drs_Bo)]{enAl = 1;}
      (junction 134) -> (junction 133) [order 2] : {enAs = 0;}
      (junction 151) -> (junction 150) [order 2] : {enAl = 0;}
      (junction 59) -> (junction 104) [order 1] : [(Ars_Do<=tol && Bl_Do<=tol)]
          | {enCr = 1;}
      (junction 116) -> (junction 126) [order 1] : [(Al_Bo<=tol && Ars_Do<=tol && ...
          | Crs_Bo<=tol && Dl_Co<=tol && ...
          | Drs_Ao<=tol && Crs_Do)]{enBl = 1;}
      (junction 59) -> (junction 104) [order 2] : {enCr = 0;}
      (junction 116) -> (junction 126) [order 2] : {enBl = 0;}
      (junction 133) -> (junction 143) [order 1] : [(Brs_Co<=tol && Dl_Co<=tol)]
          | {enAr = 1;}
      (junction 150) -> (junction 160) [order 1] : [(Bl_Do<=tol && Brs_Co<=tol ...
          | && Ars_Do<=tol && Cl_Ao<=tol ...
          | && Crs_Bo<=tol && Ars_Co)]{enDl = 1;}
      (junction 133) -> (junction 143) [order 2] : {enAr = 0;}
      (junction 150) -> (junction 160) [order 2] : {enDl = 0;}
      (junction 104) -> (junction 105) [order 1] : [(Al_Bo<=tol && Ars_Do<=tol ...
          | && Ars_Co<=tol && Cl_Ao<=tol ...
          | && Dl_Co<=tol && Drs_Ao<=tol)]
          | {enBs = 1;}
      (junction 104) -> (junction 105) [order 2] : {enBs = 0;}
      (junction 143) -> (junction 141) [order 1] : [(Bl_Do<=tol && Brs_Co<=tol ...
          | && Brs_Ao<=tol && Al_Bo<=tol ...
          | && Cl_Ao<=tol && Crs_Bo<=tol)]
          | {enDs = 1;}
      (junction 143) -> (junction 141) [order 2] : {enDs=0;}
      (junction 105) -> (junction 109) [order 1] : [Drs_Ao<=tol && Cl_Ao<=tol]
          | {enBr = 1;}
      (junction 105) -> (junction 109) [order 2] : {enBr = 0;}
      (junction 141) -> (junction 131) [order 1] : [(Crs_Bo<=tol && Al_Bo<=tol)]
          | {enDr = 1;}
      (junction 141) -> (junction 131) [order 2] : {enDr = 0;}
    timecounter -> timecounter : [after(1,sec)]{time=time+1;}
  (default) -> CompleteController : {enAl = 0; enAs = 0; enAr = 0;
      | enBl = 0; enBs = 0; enBr = 0;
      | enCl = 0; enCs = 0; enCr = 0;
      | enDl = 0; enDs = 0; enDr = 0;
      | time = 0;}
  data: Bl input; Brs input; Al input; Ars input; Cl input; Crs input; Dl input; Drs input; Al_Bo input; Ars_Do input; Ars_Co input; Bl_Do input; Brs_Co input; Brs_Ao input; Cl_Ao input; Crs_Bo input; Crs_Do input; Dl_Co input; Drs_Ao input; Drs_Bo input; enAl output =0; enAs output =0; enAr output =0; enBl output =0; enBs output =0; enBr output =0; enCl output =0; enCs output =0; enCr output =0; enDl output =0; enDs output =0; enDr output =0; green_duration_sr parameter; green_duration_l parameter; tol parameter; time output
